simulink model "signalrange01"  (Simulink 7.8)
settings: Solver=ode5  SolverMode=SingleTasking  StartTime=0.0  StopTime=10  FixedStep=0.01  RelTol=1e-3  AbsTol=1e-6
model workspace (MAT data in the model file):
  converter_data = [0  137.465208994  2.232; 0.1  137.065019157  2.075; 0.2  135.864449646  1.975; 0.3  135.664354728  1.846; 0.4  137.565256453  1.72; 0.5  140.366585312  1.564; 0.6  145.268910814  1.409; 0.7  152.872517717  1.254; 0.8  162.9773111  1.096; 0.81  164.27792807  1.08; 0.82  166.178829795  1.061; 0.83  167.979684062  1.043; 0.84  170.080680706  1.028; 0.85  172.781962105  1.012; 0.86  175.383196045  1.002; 0.87  179.585189333  1.002; 0.88  183.587087703  1.001; 0.89  189.890077635  0.998; 0.9  197.693779455  0.999; 0.92  215.902417037  1.001; 0.94  244.515990379  1.002]
  downtab = [0  5  20  35; 0  5  20  35; 0  5  25  40; 0  5  30  50; 0  30  50  80; 0  30  50  80]
  downth = [0; 5; 40; 50; 90; 100]
  emap = [-40  -44  -49  -53  -57  -61  -65  -70  -74  -78  -82; 215  117  85  66  44  29  10  -2  -13  -22  -32; 245  208  178  148  122  104  85  66  48  33  18; 264  260  241  219  193  167  152  133  119  96  85; 264  279  282  275  260  238  223  208  189  171  152; 267  290  293  297  290  275  260  256  234  212  193; 267  297  305  305  305  301  293  282  267  249  226; 267  301  308  312  319  323  319  316  297  279  253; 267  301  312  319  327  327  327  327  312  293  267; 267  301  312  319  327  334  334  334  319  305  275]
  Iei = 0.0219914882836
  nevec = [800 1200 1600 2000 2400 2800 3200 3600 4000 4400 4800]
  p0 = 0.07934
  p1 = 0.07934
  thvec = [0; 20; 30; 40; 50; 60; 70; 80; 90; 100]
  TWAIT = 2
  uptab = [10  30  50  1000000; 10  30  50  1000000; 15  30  50  1000000; 23  41  60  1000000; 40  70  100  1000000; 40  70  100  1000000]
  upth = [0; 25; 35; 50; 90; 100]
  vehicledata : num (value not decoded)
PreLoadFcn:
  | load cruise_control_data
undefined symbols (not defined in the file or in its folder): cruise_ki, cruise_kp, DiscIntNeverNeededParam, target_max, target_min, throt_max, throt_min, vel_dec, vel_inc
settings Model: DVExtractedSubsystem=cruise_control  Creator=The MathWorks Inc.  LastModifiedBy=itoy  CovMetricSettings=dcmtr  ExtModeTrigMode=oneshot  ExtModeArmWhenConnect=off  ExtModeAutoUpdateStatusClock=off
settings DataIOCC: LimitDataPoints=off  SaveOutput=off  SaveTime=off  SignalLoggingName=sigsOut
settings OptimizationCC: InlineInvariantSignals=on  InitFltsAndDblsToZero=on  EfficientMapNaN2IntZero=off
settings DebuggingCC: SignalInfNanChecking=error  SaveWithParameterizedLinksMsg=none  CheckExecutionContextPreStartOutputMsg=on  CheckExecutionContextRuntimeOutputMsg=on  SignalResolutionControl=TryResolveAll  SolverPrmCheckMsg=none  MultiTaskDSMMsg=warning  MultiTaskCondExecSysMsg=none  IntegerOverflowMsg=error  FcnCallInpInsideContextMsg=Use local settings  FrameProcessingCompatibilityMsg=none  UniqueDataStoreMsg=error  BusObjectLabelMismatch=error  RootOutportRequireBusObject=error  StrictBusMsg=ErrorOnBusTreatedAsVector  BusNameAdapt=ErrorWithoutRepair  NonBusSignalsTreatedAsBus=error
settings HardwareCC: TargetUnknown=on
settings SFSimCC: SFSimEcho=off  SimParseCustomCode=off
settings RTWCC: TLCOptions=-aAlwaysIncludeCustomSrc=1  IncludeERTFirstTime=on
settings GRTTargetCC: TargetFcnLib=ansi_tfl_tmw.mat
settings ConfigComp: Description=Design Verifier Custom Configuration Component  DVMaxTestCaseSteps=500  DVTestSuiteOptimization=CombinedObjectives (Nonlinear Extended)  DVDetectIntegerOverflow=off  DVDetectDivisionByZero=off  DVDesignMinMaxCheck=on  DVProvingStrategy=ProveWithViolationDetection

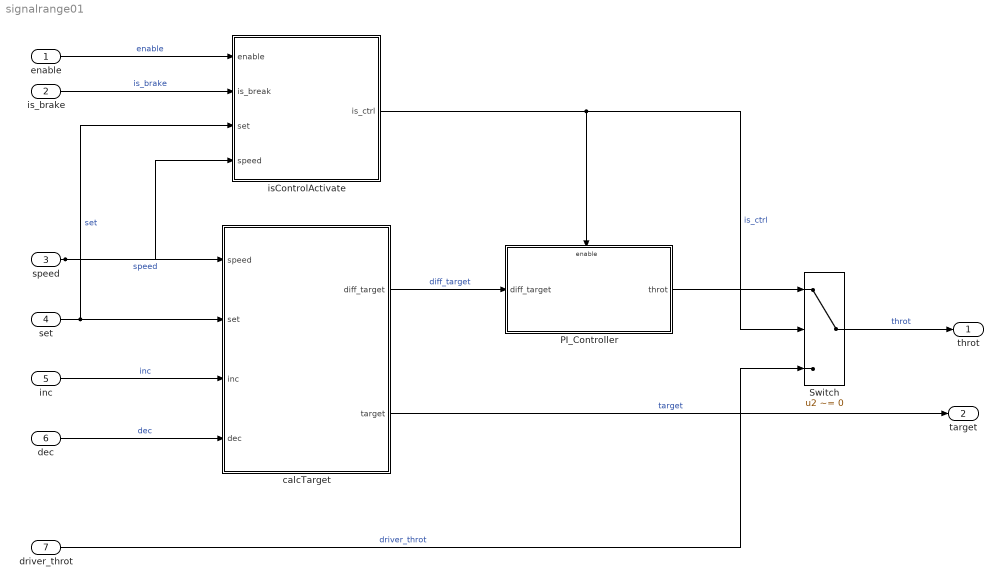
== system signalrange01 ==
  enable : Inport
  is_brake : Inport  Port=2
  speed : Inport  Port=3  OutMin=-50  OutMax=300
  set : Inport  Port=4
  inc : Inport  Port=5
  dec : Inport  Port=6
  driver_throt : Inport  Port=7
  PI_Controller : Subsystem
  Switch : Switch  Criteria=u2 ~= 0  OutDataTypeStr=Inherit: Inherit via back propagation
  calcTarget : Subsystem
  isControlActivate : Subsystem
  throt : Outport
  target : Outport  Port=2
  wires:
  isControlActivate/1(is_ctrl) -> PI_Controller/Enable, Switch/2  "is_ctrl"
  calcTarget/2(target) -> target/1  "target"
  calcTarget/1(diff_target) -> PI_Controller/1(diff_target)  "diff_target"
  dec/1 -> calcTarget/4(dec)  "dec"
  speed/1 -> calcTarget/1(speed), isControlActivate/4(speed)  "speed"
  inc/1 -> calcTarget/3(inc)  "inc"
  set/1 -> calcTarget/2(set), isControlActivate/3(set)  "set"
  Switch/1 -> throt/1  "throt"
  driver_throt/1 -> Switch/3  "driver_throt"
  is_brake/1 -> isControlActivate/2(is_break)  "is_brake"
  enable/1 -> isControlActivate/1(enable)  "enable"
  PI_Controller/1(throt) -> Switch/1

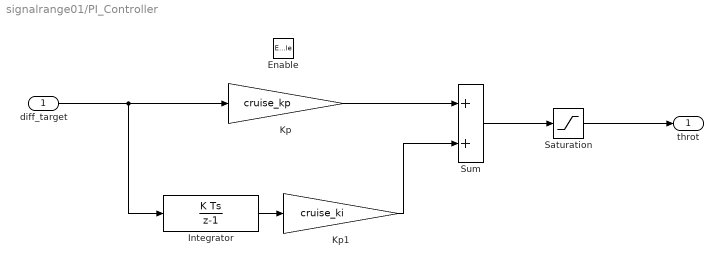
== system signalrange01/PI_Controller ==
  diff_target : Inport
  Enable : EnablePort
  Integrator : DiscreteIntegrator  gainval=1  SampleTime=-1  OutDataTypeStr=F32  UpperSaturationLimit=5  LowerSaturationLimit=-5  ICPrevOutput=DiscIntNeverNeededParam  ICPrevScaledInput=DiscIntNeverNeededParam
      settings: AttributesFormatString=<Gain = %<gainval>>
  Kp : Gain  Gain=cruise_kp  OutMin=0  OutMax=0.1  OutDataTypeStr=Inherit: Inherit via back propagation
  Kp1 : Gain  Gain=cruise_ki  ParamDataTypeStr=Inherit: Inherit from 'Gain'  OutMin=0  OutMax=0.1  OutDataTypeStr=F32
  Saturation : Saturate  UpperLimit=throt_max  LowerLimit=throt_min  OutDataTypeStr=Inherit: Inherit via back propagation
      settings: AttributesFormatString=<UpperLimit = %<UpperLimit>>\n<LowerLimit = %<LowerLimit>>
  Sum : Sum  AccumDataTypeStr=F32  OutDataTypeStr=F32
  throt : Outport
  wires:
  Sum/1 -> Saturation/1
  diff_target/1 -> Integrator/1, Kp/1
  Integrator/1 -> Kp1/1
  Kp/1 -> Sum/1
  Saturation/1 -> throt/1
  Kp1/1 -> Sum/2

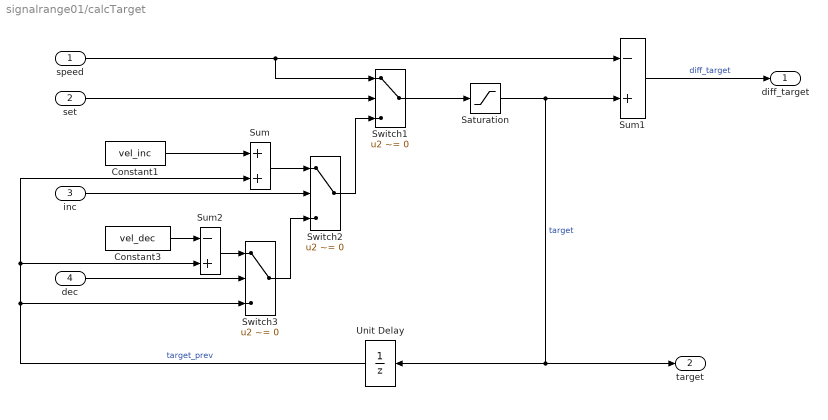
== system signalrange01/calcTarget ==
  speed : Inport
  set : Inport  Port=2
  inc : Inport  Port=3
  dec : Inport  Port=4
  Constant1 : Constant  Value=vel_inc
  Constant3 : Constant  Value=vel_dec
  Saturation : Saturate  UpperLimit=target_max  LowerLimit=target_min
      settings: AttributesFormatString=<UpperLimit = %<UpperLimit>>\n<LowerLimit = %<LowerLimit>>
  Sum : Sum
  Sum1 : Sum  Inputs=-+  OutDataTypeStr=Inherit: Same as first input
  Sum2 : Sum  Inputs=-+
  Switch1 : Switch  Criteria=u2 ~= 0
  Switch2 : Switch  Criteria=u2 ~= 0
  Switch3 : Switch  Criteria=u2 ~= 0
  Unit Delay : UnitDelay  SampleTime=-1
  diff_target : Outport
  target : Outport  Port=2
  wires:
  Sum1/1 -> diff_target/1  "diff_target"
  Switch1/1 -> Saturation/1
  Unit Delay/1 -> Sum/2, Sum2/2, Switch3/3  "target_prev"
  Switch3/1 -> Switch2/3
  Switch2/1 -> Switch1/3
  Sum2/1 -> Switch3/1
  Constant3/1 -> Sum2/1
  dec/1 -> Switch3/2
  Sum/1 -> Switch2/1
  Constant1/1 -> Sum/1
  inc/1 -> Switch2/2
  speed/1 -> Sum1/1, Switch1/1
  set/1 -> Switch1/2
  Saturation/1 -> Unit Delay/1, target/1, Sum1/2  "target"

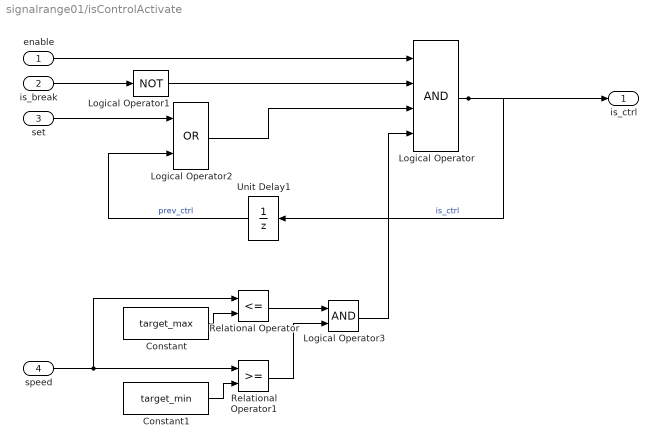
== system signalrange01/isControlActivate ==
  enable : Inport
  is_break : Inport  Port=2
  set : Inport  Port=3
  speed : Inport  Port=4
  Constant : Constant  Value=target_max
  Constant1 : Constant  Value=target_min
  Logical Operator : Logic  Inputs=4  AllPortsSameDT=off  OutDataTypeStr=boolean
  Logical Operator1 : Logic  Operator=NOT  AllPortsSameDT=off  OutDataTypeStr=boolean
  Logical Operator2 : Logic  Operator=OR  AllPortsSameDT=off  OutDataTypeStr=boolean
  Logical Operator3 : Logic  AllPortsSameDT=off  OutDataTypeStr=boolean
  Relational Operator : RelationalOperator  Operator=<=  OutDataTypeStr=boolean
  Relational Operator1 : RelationalOperator  OutDataTypeStr=boolean
  Unit Delay1 : UnitDelay  SampleTime=-1
  is_ctrl : Outport
  wires:
  Logical Operator/1 -> Unit Delay1/1, is_ctrl/1  "is_ctrl"
  Unit Delay1/1 -> Logical Operator2/2  "prev_ctrl"
  Logical Operator2/1 -> Logical Operator/3
  Logical Operator1/1 -> Logical Operator/2
  set/1 -> Logical Operator2/1
  enable/1 -> Logical Operator/1
  is_break/1 -> Logical Operator1/1
  Constant1/1 -> Relational Operator1/2
  speed/1 -> Relational Operator1/1, Relational Operator/1
  Relational Operator/1 -> Logical Operator3/1
  Relational Operator1/1 -> Logical Operator3/2
  Logical Operator3/1 -> Logical Operator/4
  Constant/1 -> Relational Operator/2
